simulink model "Copy_2_of_signal_injection"  (R2023a)
settings: Solver=FixedStepAuto  StartTime=0.0  StopTime=10/fsw  FixedStep=1e-7  RelTol=1e-3
InitFcn:
  | f_fund=50;
  | ma=1;
  | fsw=100e3;
settings Model: Creator=enesa  LastModifiedBy=enesa

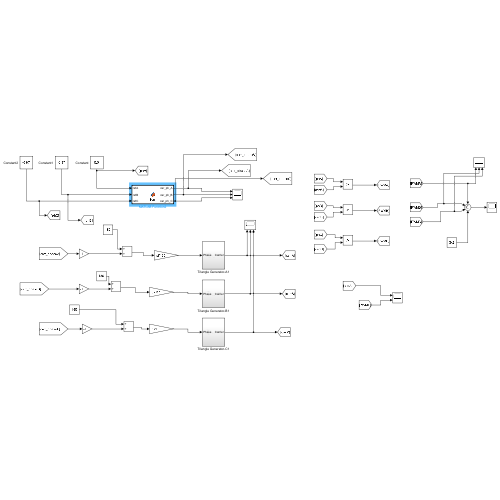
[thumbnail: Simulink's stored preview of the top-level diagram]
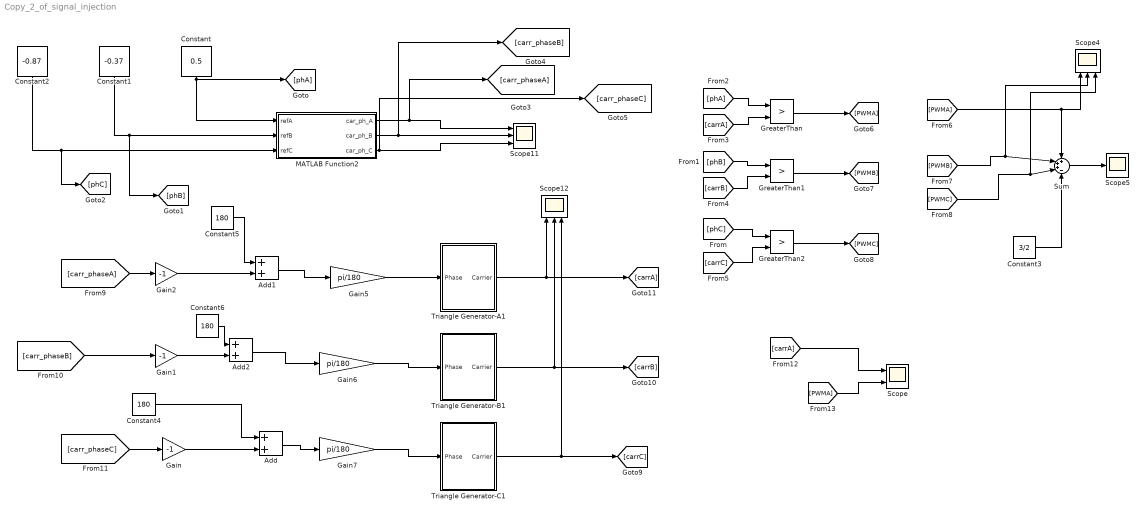
== system Copy_2_of_signal_injection ==
  Add : Sum
  Add1 : Sum
  Add2 : Sum
  Constant : Constant  Value=0.5  VectorParams1D=off  SampleTime=-1
  Constant1 : Constant  Value=-0.37  VectorParams1D=off  SampleTime=-1
  Constant2 : Constant  Value=-0.87  VectorParams1D=off  SampleTime=-1
  Constant3 : Constant  Value=3/2
  Constant4 : Constant  Value=180
  Constant5 : Constant  Value=180
  Constant6 : Constant  Value=180
  Gain : Gain  Gain=-1
  Gain1 : Gain  Gain=-1
  Gain2 : Gain  Gain=-1
  Gain5 : Gain  Gain=pi/180
  Gain6 : Gain  Gain=pi/180
  Gain7 : Gain  Gain=pi/180
  GreaterThan : RelationalOperator  Operator=>  OutDataTypeStr=boolean  RndMeth=Simplest  InputSameDT=off
  GreaterThan1 : RelationalOperator  Operator=>  OutDataTypeStr=boolean  RndMeth=Simplest  InputSameDT=off
  GreaterThan2 : RelationalOperator  Operator=>  OutDataTypeStr=boolean  RndMeth=Simplest  InputSameDT=off
  MATLAB Function2 : MATLAB Function  TreatAsAtomicUnit=on
  Scope : Scope  NumInputPorts=2
  Scope11 : Scope  NumInputPorts=3
  Scope12 : Scope  NumInputPorts=3
  Scope4 : Scope  NumInputPorts=3
  Scope5 : Scope
  Sum : Sum  Inputs=+++-
  Triangle Generator-A1 : Subsystem
  Triangle Generator-B1 : Subsystem
  Triangle Generator-C1 : Subsystem
  wires:
  [phA] -> GreaterThan/1
  [carrA] -> GreaterThan/2
  [phB] -> GreaterThan1/1
  [carrB] -> GreaterThan1/2
  [phC] -> GreaterThan2/1
  [carrC] -> GreaterThan2/2
  GreaterThan/1 -> [PWMA]
  GreaterThan1/1 -> [PWMB]
  GreaterThan2/1 -> [PWMC]
  [PWMA] -> Sum/1, Scope4/1
  [PWMB] -> Sum/2, Scope4/2
  [PWMC] -> Sum/3, Scope4/3
  Sum/1 -> Scope5/1
  Constant3/1 -> Sum/4
  MATLAB Function2/1(car_ph_A) -> [carr_phaseA], Scope11/1
  MATLAB Function2/2(car_ph_B) -> [carr_phaseB], Scope11/2
  Triangle Generator-A1/1(Carrier) -> Scope12/1, [carrA]
  Gain7/1 -> Triangle Generator-C1/1(Phase)
  Gain6/1 -> Triangle Generator-B1/1(Phase)
  Triangle Generator-B1/1(Carrier) -> [carrB], Scope12/2
  Triangle Generator-C1/1(Carrier) -> [carrC], Scope12/3
  Constant/1 -> MATLAB Function2/1(refA), [phA]
  Constant2/1 -> [phC], MATLAB Function2/3(refC)
  Gain5/1 -> Triangle Generator-A1/1(Phase)
  Constant1/1 -> [phB], MATLAB Function2/2(refB)
  [carr_phaseA] -> Gain2/1
  MATLAB Function2/3(car_ph_C) -> [carr_phaseC], Scope11/3
  [carr_phaseC] -> Gain/1
  Constant4/1 -> Add/1
  Constant5/1 -> Add1/1
  [carrA] -> Scope/1
  [PWMA] -> Scope/2
  [carr_phaseB] -> Gain1/1
  Constant6/1 -> Add2/1
  Gain/1 -> Add/2
  Gain1/1 -> Add2/2
  Gain2/1 -> Add1/2
  Add2/1 -> Gain6/1
  Add/1 -> Gain7/1
  Add1/1 -> Gain5/1

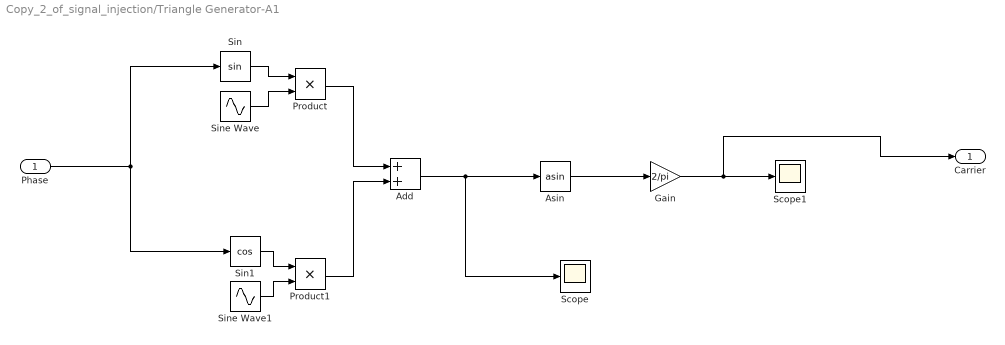
== system Copy_2_of_signal_injection/Triangle Generator-A1 ==
  Phase : Inport
  Add : Sum
  Asin : Trigonometry  Operator=asin
  Gain : Gain  Gain=2/pi
  Product : Product
  Product1 : Product
  Scope : Scope
  Scope1 : Scope
  Sin : Trigonometry
  Sin1 : Trigonometry  Operator=cos
  Sine Wave : Sin  Frequency=2*pi*fsw  SampleTime=0
  Sine Wave1 : Sin  Frequency=2*pi*fsw  Phase=-pi/2  SampleTime=0
  Carrier : Outport
  wires:
  Sin/1 -> Product/1
  Sine Wave/1 -> Product/2
  Phase/1 -> Sin/1, Sin1/1
  Product/1 -> Add/1
  Asin/1 -> Gain/1
  Gain/1 -> Carrier/1, Scope1/1
  Sine Wave1/1 -> Product1/2
  Product1/1 -> Add/2
  Add/1 -> Asin/1, Scope/1
  Sin1/1 -> Product1/1

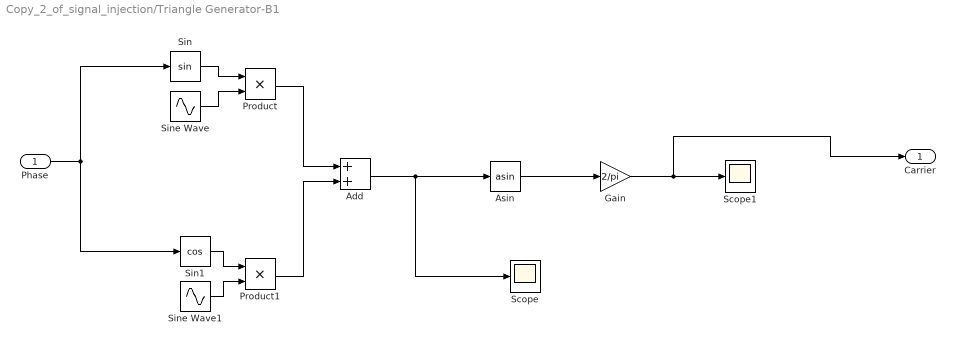
== system Copy_2_of_signal_injection/Triangle Generator-B1 ==
  Phase : Inport
  Add : Sum
  Asin : Trigonometry  Operator=asin
  Gain : Gain  Gain=2/pi
  Product : Product
  Product1 : Product
  Scope : Scope
  Scope1 : Scope
  Sin : Trigonometry
  Sin1 : Trigonometry  Operator=cos
  Sine Wave : Sin  Frequency=2*pi*fsw  SampleTime=0
  Sine Wave1 : Sin  Frequency=2*pi*fsw  Phase=-pi/2  SampleTime=0
  Carrier : Outport
  wires:
  Sin/1 -> Product/1
  Sine Wave/1 -> Product/2
  Phase/1 -> Sin1/1, Sin/1
  Product/1 -> Add/1
  Asin/1 -> Gain/1
  Gain/1 -> Carrier/1, Scope1/1
  Sine Wave1/1 -> Product1/2
  Product1/1 -> Add/2
  Add/1 -> Asin/1, Scope/1
  Sin1/1 -> Product1/1

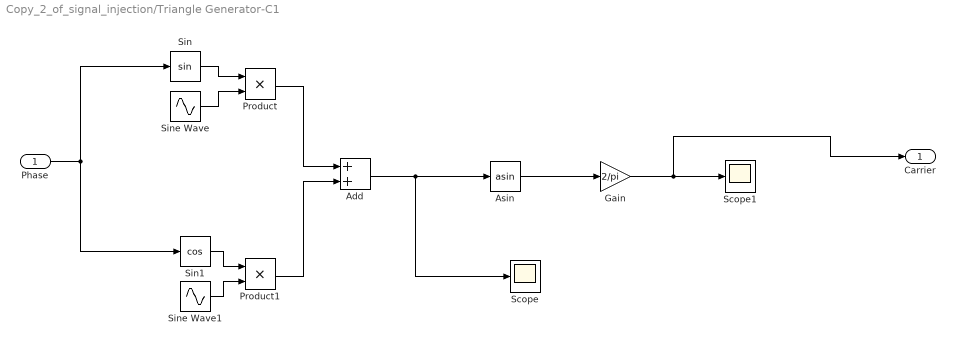
== system Copy_2_of_signal_injection/Triangle Generator-C1 ==
  Phase : Inport
  Add : Sum
  Asin : Trigonometry  Operator=asin
  Gain : Gain  Gain=2/pi
  Product : Product
  Product1 : Product
  Scope : Scope
  Scope1 : Scope
  Sin : Trigonometry
  Sin1 : Trigonometry  Operator=cos
  Sine Wave : Sin  Frequency=2*pi*fsw  SampleTime=0
  Sine Wave1 : Sin  Frequency=2*pi*fsw  Phase=-pi/2  SampleTime=0
  Carrier : Outport
  wires:
  Sin/1 -> Product/1
  Sine Wave/1 -> Product/2
  Phase/1 -> Sin1/1, Sin/1
  Product/1 -> Add/1
  Asin/1 -> Gain/1
  Gain/1 -> Carrier/1, Scope1/1
  Sine Wave1/1 -> Product1/2
  Product1/1 -> Add/2
  Add/1 -> Asin/1, Scope/1
  Sin1/1 -> Product1/1

== matlab function Copy_2_of_signal_injection/MATLAB Function2 ==
  data: refA input; car_ph_A output; refB input; refC input; car_ph_B output; car_ph_C output
function [car_ph_A, car_ph_B, car_ph_C]= fcn(refA, refB, refC)

refA2=(1+refA)/2;
refB2=(1+refB)/2;
refC2=(1+refC)/2,


car_ph_B=0;
car_ph_A=360*(refB2+refA2-2*refC2)/2
car_ph_C=360*(-refB2+refC2)/2;



end
